simulink model "sampleModel1585_5_sub_sub"  (R2023a)
settings: Solver=VariableStepAuto  StartTime=0.0  StopTime=10.0  RelTol=1e-3
libraries: hdlsllib x7, simulink x1
settings Model: Creator=user1  LastModifiedBy=user1

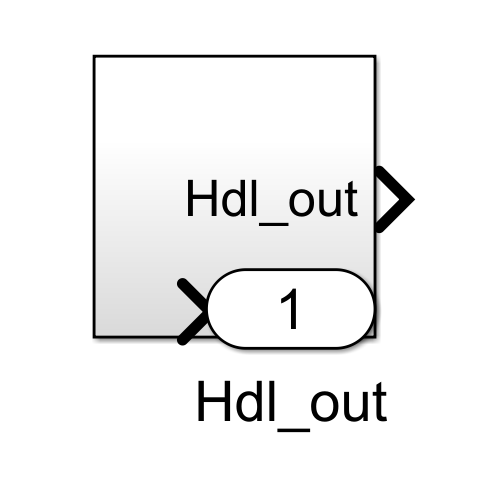
[thumbnail: Simulink's stored preview of the top-level diagram]
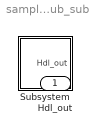
== system sampleModel1585_5_sub_sub ==
  Subsystem : Subsystem
  Hdl_out : Outport  OutDataTypeStr=uint8

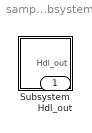
== system sampleModel1585_5_sub_sub/Subsystem ==
  Subsystem : Subsystem
  Hdl_out : Outport  OutDataTypeStr=uint8

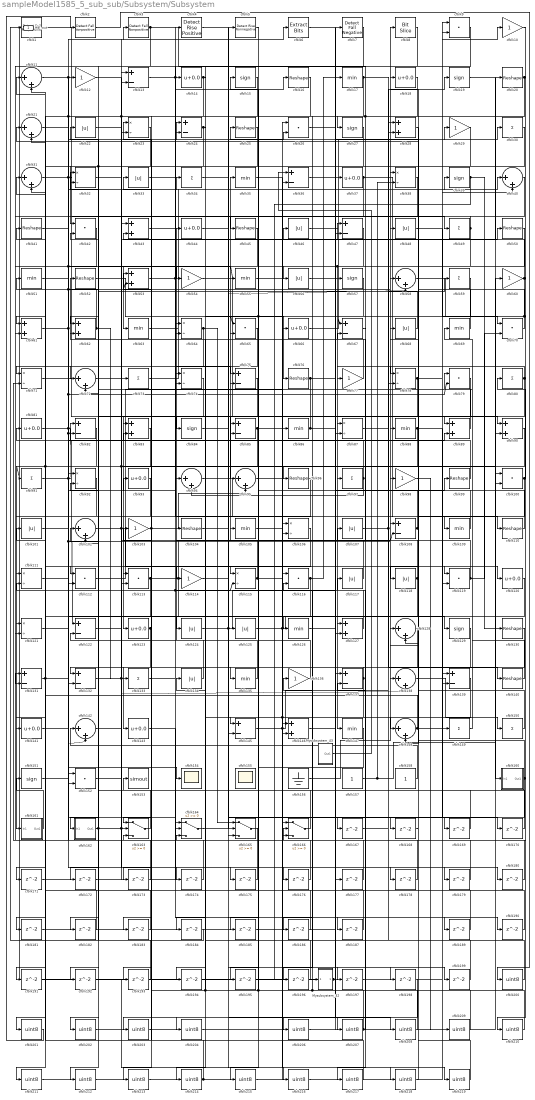
== system sampleModel1585_5_sub_sub/Subsystem/Subsystem ==
  Mysubsystem_32 : Subsystem  TreatAsAtomicUnit=on  RTWFcnName=Mysubsystem_32
      settings: RTWFcnNameOpts=User specified  RTWFileNameOpts=Use function name
  Mysubsystem_43 : Subsystem  TreatAsAtomicUnit=on  RTWFcnName=Mysubsystem_43
      settings: RTWFcnNameOpts=User specified  RTWFileNameOpts=Use function name
  cfblk1 : hdlsllib/Logic and Bit Operations/Detect Fall Nonpositive  vinit=0  OutDataTypeStr=uint8
  cfblk{10,12,29,54,60,77,98,103,114,136} (10 alike) : Gain  OutDataTypeStr=uint8
  cfblk{9,26,42,65,70,79,100,112..113,116,119,152} (12 alike) : DotProduct  OutDataTypeStr=uint8
  cfblk{22,33,46,48,56,68,101,107,117..118,124..125,134} (13 alike) : Abs  OutDataTypeStr=uint8  SaturateOnIntegerOverflow=off
  cfblk{11,21,31,40,58,72,94..95,102,128,138,142,148} (13 alike) : Sum  Inputs=|++  OutDataTypeStr=uint8
  cfblk{16,20,25,41,45,50,52,76,96,99,104,110,130,140} (14 alike) : Reshape
  cfblk{17,35,51,55,63,69,86,88,105,109,126,135,147} (13 alike) : MinMax  OutDataTypeStr=uint8
  cfblk{23,32,38,64,71,74,78,87,92,106,111,115,121} (13 alike) : Product  Inputs=*/  OutDataTypeStr=uint8  RndMeth=Zero  SaturateOnIntegerOverflow=on
  cfblk{13,24,36,47,67,75,82,85,108,122,131..132,137,139,145} (15 alike) : Sum  Inputs=+-  OutDataTypeStr=uint8
  cfblk{14,18,37,44,66,81,93,120,123,141,143} (11 alike) : Bias  Bias=0.0  SaturateOnIntegerOverflow=off
  cfblk{28,43,53,61..62,83,89..90,127,146} (10 alike) : Sum  OutDataTypeStr=uint8
  cfblk{15,19,27,39,57,84,129,151} (8 alike) : Signum
  cfblk{30,34,49,59,73,80,91,97,133,149..150} (11 alike) : Sum  Inputs=+  OutDataTypeStr=uint8
  cfblk153 : ToWorkspace  VariableName=simout  SaveFormat=Timeseries  SampleTime=-1
  cfblk154 : Scope
  cfblk155 : Scope
      settings: Floating=on
  cfblk156 : Ground
  cfblk157 : Constant  OutDataTypeStr=uint8  SampleTime=-1
  cfblk158 : Constant  OutDataTypeStr=uint8  SampleTime=-1
  cfblk160 : Subsystem
      settings: LibrarySourceBlock=|
      | hdlsllib/Ports &
      | Subsystems/Subsystem
  cfblk161 : Subsystem
      settings: LibrarySourceBlock=|
      | hdlsllib/Ports &
      | Subsystems/Subsystem
  cfblk162 : Subsystem
      settings: LibrarySourceBlock=|
      | hdlsllib/Ports &
      | Subsystems/Subsystem
  cfblk{163..166} (4 alike) : Switch  OutDataTypeStr=uint8  SaturateOnIntegerOverflow=off  InputSameDT=off
  cfblk{167..187,189..199} (32 alike) : Delay  SampleTime=1
  cfblk2 : hdlsllib/Logic and Bit Operations/Detect Fall Nonpositive  vinit=0  OutDataTypeStr=uint8
  cfblk{200..204,206..219} (19 alike) : DataTypeConversion  OutDataTypeStr=uint8  SaturateOnIntegerOverflow=off  RndMeth=Floor
  cfblk3 : hdlsllib/Logic and Bit Operations/Detect Fall Nonpositive  vinit=0  OutDataTypeStr=uint8
  cfblk4 : hdlsllib/Logic and Bit Operations/Detect Rise Positive  vinit=0  OutDataTypeStr=uint8
  cfblk5 : hdlsllib/Logic and Bit Operations/Detect Rise Nonnegative  vinit=0  OutDataTypeStr=uint8
  cfblk6 : simulink/Logic and Bit Operations/Extract Bits  bitsToExtract=Upper half  numBits=8  bitIdxRange=[0 7]  outScalingMode=Preserve fixed-point scaling
      settings: LibrarySourceBlock=|
      | hdlsllib/Logic and Bit
      | Operations/Extract Bits
  cfblk7 : hdlsllib/Logic and Bit Operations/Detect Fall Negative  vinit=0  OutDataTypeStr=uint8
  cfblk8 : hdlsllib/Logic and Bit Operations/Bit Slice  lidx=7  ridx=0
  Hdl_out : Outport  OutDataTypeStr=uint8
  wires:
  Mysubsystem_43/1(Out1) -> cfblk36/1
  Mysubsystem_32/1(Out1) -> cfblk9/1, Hdl_out/1
  cfblk219/1 -> cfblk128/2
  cfblk194/1 -> cfblk219/1
  cfblk218/1 -> cfblk128/1
  cfblk35/1 -> cfblk218/1
  cfblk217/1 -> cfblk81/1
  cfblk128/1 -> cfblk217/1
  cfblk216/1 -> cfblk139/2
  cfblk192/1 -> cfblk216/1
  cfblk215/1 -> cfblk139/1
  cfblk120/1 -> cfblk215/1
  cfblk214/1 -> cfblk103/1, cfblk166/1
  cfblk213/1 -> cfblk106/2
  cfblk198/1 -> cfblk213/1
  cfblk212/1 -> cfblk106/1
  cfblk74/1 -> cfblk212/1
  cfblk211/1 -> cfblk116/1
  cfblk106/1 -> cfblk211/1
  cfblk210/1 -> cfblk98/1
  cfblk209/1 -> cfblk83/2, cfblk104/1, cfblk136/1
  cfblk208/1 -> cfblk105/1
  cfblk26/1 -> cfblk208/1
  cfblk207/1 -> cfblk65/2, cfblk163/3, cfblk117/1
  cfblk206/1 -> cfblk9/2
  cfblk4/1 -> cfblk206/1
  cfblk204/1 -> cfblk60/1
  cfblk9/1 -> cfblk204/1
  cfblk203/1 -> cfblk7/1
  cfblk129/1 -> cfblk203/1
  cfblk202/1 -> cfblk66/1
  cfblk7/1 -> cfblk202/1
  cfblk201/1 -> cfblk2/1
  cfblk200/1 -> cfblk134/1
  cfblk2/1 -> cfblk200/1
  cfblk199/1 -> cfblk28/1
  cfblk126/1 -> cfblk199/1
  cfblk84/1 -> cfblk198/1
  cfblk197/1 -> cfblk119/2
  cfblk196/1 -> cfblk164/3
  cfblk195/1 -> cfblk47/2
  cfblk147/1 -> cfblk195/1
  cfblk59/1 -> cfblk194/1
  cfblk193/1 -> cfblk122/2
  cfblk27/1 -> cfblk193/1
  cfblk191/1 -> cfblk26/1
  cfblk83/1 -> cfblk191/1
  cfblk190/1 -> cfblk62/2
  cfblk189/1 -> cfblk137/2
  cfblk143/1 -> cfblk189/1
  cfblk187/1 -> cfblk116/2
  cfblk44/1 -> cfblk187/1
  cfblk186/1 -> cfblk142/1
  cfblk57/1 -> cfblk186/1
  cfblk185/1 -> cfblk166/3
  cfblk184/1 -> cfblk1/1
  cfblk183/1 -> cfblk11/1
  cfblk182/1 -> cfblk21/2
  cfblk181/1 -> cfblk87/2
  cfblk180/1 -> cfblk164/1
  cfblk95/1 -> cfblk180/1
  cfblk179/1 -> cfblk102/2
  cfblk178/1 -> cfblk131/1
  cfblk114/1 -> cfblk178/1
  cfblk177/1 -> cfblk152/1
  cfblk6/1 -> cfblk177/1
  cfblk176/1 -> cfblk92/2
  cfblk175/1 -> cfblk31/1
  cfblk22/1 -> cfblk175/1
  cfblk174/1 -> cfblk72/2
  cfblk173/1 -> cfblk13/1
  cfblk75/1 -> cfblk173/1
  cfblk172/1 -> cfblk43/1
  cfblk40/1 -> cfblk172/1
  cfblk171/1 -> cfblk74/2
  cfblk170/1 -> cfblk64/1
  cfblk169/1 -> cfblk42/2
  cfblk36/1 -> cfblk169/1
  cfblk168/1 -> cfblk138/1
  cfblk34/1 -> cfblk168/1
  cfblk167/1 -> cfblk78/2
  cfblk67/1 -> cfblk167/1
  cfblk119/1 -> cfblk67/2, cfblk70/2
  cfblk65/1 -> cfblk141/1
  cfblk115/1 -> cfblk64/2, cfblk50/1
  cfblk76/1 -> cfblk95/1, cfblk30/1
  cfblk149/1 -> cfblk79/1
  cfblk104/1 -> cfblk125/1
  cfblk151/1 -> cfblk38/1
  cfblk56/1 -> cfblk89/1
  cfblk33/1 -> cfblk16/1
  cfblk92/1 -> cfblk152/2
  cfblk107/1 -> cfblk120/1, cfblk59/1
  cfblk53/1 -> cfblk4/1, cfblk75/1
  cfblk58/1 -> cfblk100/1
  cfblk111/1 -> cfblk88/1
  cfblk148/1 -> cfblk111/2, cfblk40/2
  cfblk28/1 -> cfblk78/1
  cfblk121/1 -> cfblk108/2, cfblk93/1
  cfblk48/1 -> cfblk70/1
  cfblk158/1 -> cfblk32/2
  cfblk72/1 -> cfblk138/2, cfblk100/2
  cfblk8/1 -> cfblk24/2
  cfblk16/1 -> cfblk23/2
  cfblk131/1 -> cfblk34/1, cfblk79/2, cfblk41/1
  cfblk123/1 -> cfblk163/1, cfblk182/1
  cfblk127/1 -> cfblk101/1
  cfblk21/1 -> cfblk142/2, cfblk55/1
  cfblk42/1 -> cfblk131/2
  cfblk145/1 -> cfblk19/1, cfblk197/1
  cfblk150/1 -> cfblk25/1
  cfblk163/1 -> cfblk153/1
  cfblk47/1 -> cfblk62/1
  cfblk102/1 -> cfblk119/1, cfblk94/1
  cfblk52/1 -> cfblk76/1
  cfblk32/1 -> cfblk26/2
  cfblk51/1 -> cfblk164/2, cfblk53/2
  cfblk64/1 -> cfblk72/1, cfblk165/1
  cfblk12/1 -> cfblk49/1
  cfblk124/1 -> cfblk37/1, cfblk58/2
  cfblk77/1 -> cfblk52/1
  cfblk71/1 -> cfblk113/1
  cfblk110/1 -> cfblk43/2
  cfblk41/1 -> cfblk92/1
  cfblk55/1 -> cfblk86/1
  cfblk62/1 -> cfblk31/2, cfblk133/1
  cfblk11/1 -> cfblk54/1
  cfblk166/1 -> cfblk53/1
  cfblk89/1 -> cfblk51/1
  cfblk91/1 -> cfblk57/1, cfblk163/2
  cfblk100/1 -> cfblk148/2, cfblk80/1
  cfblk96/1 -> cfblk111/1
  cfblk30/1 -> cfblk118/1
  cfblk70/1 -> cfblk67/1, cfblk21/1
  cfblk140/1 -> cfblk69/1
  cfblk133/1 -> cfblk48/1, cfblk115/2
  cfblk165/1 -> cfblk71/2
  cfblk113/1 -> cfblk108/1, cfblk146/1, cfblk132/2
  cfblk157/1 -> cfblk90/2, cfblk38/2
  cfblk54/1 -> cfblk90/1
  cfblk97/1 -> cfblk11/2, cfblk94/2
  cfblk142/1 -> cfblk46/1
  cfblk60/1 -> cfblk65/1, cfblk185/1, cfblk23/1
  cfblk15/1 -> cfblk91/1, cfblk201/1
  cfblk5/1 -> cfblk145/1
  cfblk101/1 -> cfblk24/1
  cfblk43/1 -> cfblk74/1
  cfblk68/1 -> cfblk32/1
  cfblk88/1 -> cfblk170/1, cfblk171/1
  cfblk79/1 -> cfblk112/1
  cfblk17/1 -> cfblk140/1, cfblk83/1
  cfblk152/1 -> cfblk13/2
  cfblk23/1 -> cfblk132/1, cfblk61/1
  cfblk38/1 -> cfblk162/1(In1)
  cfblk63/1 -> cfblk20/1
  cfblk90/1 -> cfblk115/1
  cfblk164/1 -> cfblk5/1
  cfblk87/1 -> cfblk28/2
  cfblk160/1(Out1) -> cfblk18/1, cfblk165/3
  cfblk112/1 -> cfblk36/2
  cfblk61/1 -> cfblk82/2, cfblk179/1, cfblk58/1
  cfblk78/1 -> cfblk124/1, cfblk10/1
  cfblk29/1 -> cfblk56/1
  cfblk122/1 -> cfblk107/1
  cfblk18/1 -> cfblk97/1, cfblk196/1
  cfblk14/1 -> cfblk71/1, cfblk112/2, cfblk113/2, cfblk114/1
  cfblk161/1(Out1) -> cfblk151/1
  cfblk103/1 -> cfblk33/1, cfblk95/2
  cfblk132/1 -> cfblk73/1, cfblk174/1
  cfblk19/1 -> cfblk160/1(In1)
  cfblk94/1 -> cfblk149/1
  cfblk69/1 -> cfblk47/1
  cfblk105/1 -> cfblk207/1
  cfblk85/1 -> cfblk121/1, cfblk127/2
  cfblk24/1 -> cfblk183/1, cfblk184/1
  cfblk99/1 -> cfblk82/1
  cfblk138/1 -> cfblk150/1
  cfblk162/1(Out1) -> cfblk6/1, cfblk176/1, cfblk22/1
  cfblk125/1 -> cfblk129/1, cfblk190/1
  cfblk31/1 -> cfblk137/1, cfblk154/1
  cfblk137/1 -> cfblk146/2, cfblk145/2, cfblk135/1
  cfblk136/1 -> cfblk15/1
  cfblk135/1 -> cfblk102/1
  cfblk109/1 -> cfblk68/1
  cfblk81/1 -> cfblk122/1, cfblk127/1
  cfblk66/1 -> cfblk39/1
  cfblk20/1 -> cfblk165/2, cfblk210/1
  cfblk80/1 -> cfblk77/1, cfblk96/1
  cfblk118/1 -> cfblk85/2, cfblk181/1
  cfblk37/1 -> cfblk110/1, cfblk121/2
  cfblk45/1 -> cfblk63/1
  cfblk49/1 -> cfblk45/1, cfblk192/1
  cfblk108/1 -> cfblk148/1, cfblk75/2
  cfblk86/1 -> cfblk84/1, cfblk89/2
  cfblk3/1 -> cfblk27/1, cfblk61/2
  cfblk117/1 -> cfblk35/1
  cfblk141/1 -> cfblk12/1, cfblk3/1
  cfblk130/1 -> cfblk143/1
  cfblk93/1 -> cfblk123/1
  cfblk13/1 -> cfblk14/1, cfblk109/1
  cfblk25/1 -> cfblk42/1
  cfblk98/1 -> cfblk209/1
  cfblk134/1 -> cfblk44/1
  cfblk73/1 -> cfblk40/1
  cfblk156/1 -> cfblk8/1
  cfblk46/1 -> cfblk29/1
  cfblk10/1 -> cfblk166/2
  cfblk1/1 -> cfblk87/1
  cfblk116/1 -> cfblk17/1, cfblk126/1
  cfblk146/1 -> cfblk99/1
  cfblk139/1 -> cfblk214/1
  cfblk82/1 -> cfblk161/1(In1)
  cfblk50/1 -> cfblk147/1, cfblk85/1
  cfblk39/1 -> Mysubsystem_32/1(In1), cfblk130/1

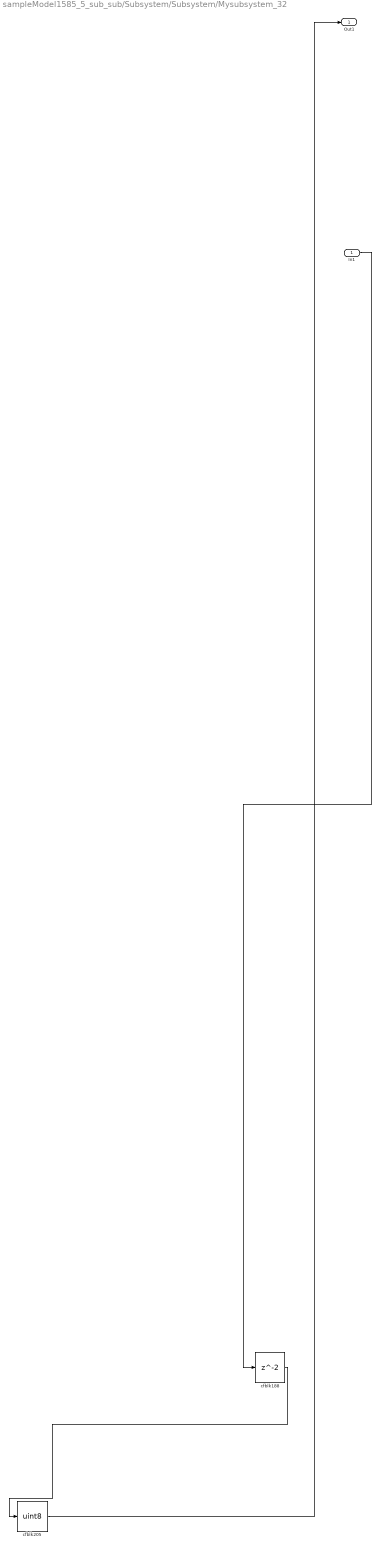
== system sampleModel1585_5_sub_sub/Subsystem/Subsystem/Mysubsystem_32 ==
  In1 : Inport
  cfblk188 : Delay  SampleTime=1
  cfblk205 : DataTypeConversion  OutDataTypeStr=uint8  SaturateOnIntegerOverflow=off  RndMeth=Floor
  Out1 : Outport
  wires:
  cfblk188/1 -> cfblk205/1
  In1/1 -> cfblk188/1
  cfblk205/1 -> Out1/1

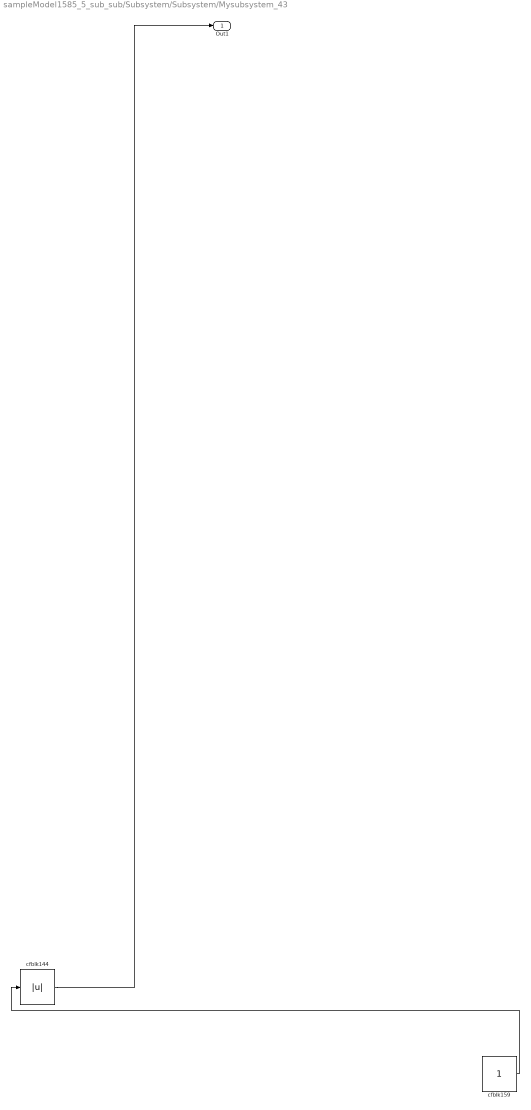
== system sampleModel1585_5_sub_sub/Subsystem/Subsystem/Mysubsystem_43 ==
  cfblk144 : Abs  SaturateOnIntegerOverflow=off
  cfblk159 : Constant  SampleTime=-1
  Out1 : Outport
  wires:
  cfblk159/1 -> cfblk144/1
  cfblk144/1 -> Out1/1

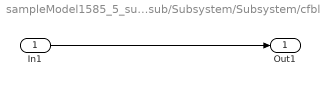
== system sampleModel1585_5_sub_sub/Subsystem/Subsystem/cfblk160 ==
  In1 : Inport
  Out1 : Outport
  wires:
  In1/1 -> Out1/1

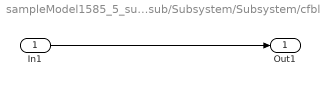
== system sampleModel1585_5_sub_sub/Subsystem/Subsystem/cfblk161 ==
  In1 : Inport
  Out1 : Outport
  wires:
  In1/1 -> Out1/1

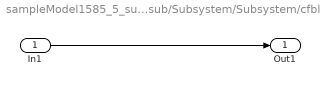
== system sampleModel1585_5_sub_sub/Subsystem/Subsystem/cfblk162 ==
  In1 : Inport
  Out1 : Outport
  wires:
  In1/1 -> Out1/1
